simulink model "sim1"  (R2020a)
settings: Solver=ode4  StartTime=0.0  StopTime=inf  FixedStep=0.001  RelTol=1e-3
undefined symbols (not defined in the file or in its folder): National_Instruments, PCI
libraries: sldrtlib x3
settings Model: SimulationMode=external  ExtModeTrigDuration=60000  ExtModeArchiveMode=auto  ExtModeArchiveFileName=data  ExtModeArchiveDirName=E:\work\me-clab2\Lab01  ExtModeAddSuffixToVar=on  Creator=me-clab2  LastModifiedBy=me-clab2
settings RTWCC: Description=Simulink Desktop Real-Time  SystemTargetFile=sldrt.tlc  TemplateMakefile=sldrt.tmf  RTWCompilerOptimization=on
settings CodeAppCC: MaxIdLength=95
settings SimulinkDesktopRealTimeCC: TargetPreCompLibLocation=C:\Program Files\MATLAB\R2020a\toolbox\sldrt\lib\win64

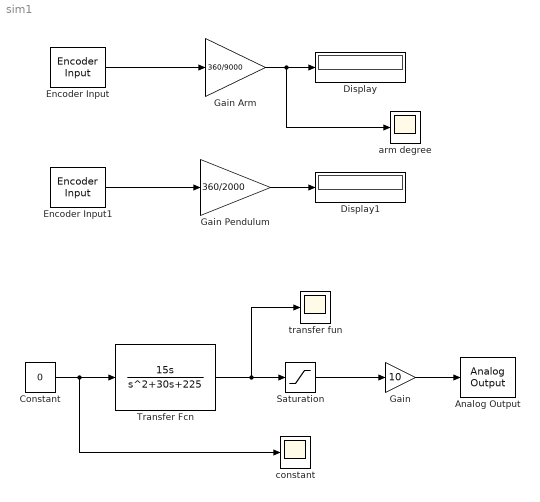
== system sim1 ==
  Analog Output : sldrtlib/Analog Output  SampleTime=0.001  MaxMissedTicks=10  ShowMissedTicks=off  YieldWhenWaiting=off  DrvName=National_Instruments/PCI-6221  DrvAddress=4294967295  DrvOptions=[0 0 0 2 2]  Channels=[2]  RangeMode=1  VoltRange=1  InitialValue=0  FinalValue=0
      settings: AttributesFormatString=National Instruments\nPCI-6221 [auto]
  Constant : Constant  Value=0
  Display : Display
  Display1 : Display
  Encoder Input : sldrtlib/Encoder Input  SampleTime=0.001  MaxMissedTicks=10  ShowMissedTicks=off  YieldWhenWaiting=off  DrvName=National_Instruments/PCI-6221  DrvAddress=4294967295  DrvOptions=[0 0 0 2 2]  Channels=[1]  QuadMode=3  IndexPulse=1  InputFilter=Inf  DataType=1
      settings: AttributesFormatString=National Instruments\nPCI-6221 [auto]
  Encoder Input1 : sldrtlib/Encoder Input  SampleTime=0.001  MaxMissedTicks=10  ShowMissedTicks=off  YieldWhenWaiting=off  DrvName=National_Instruments/PCI-6221  DrvAddress=4294967295  DrvOptions=[0 0 0 2 2]  Channels=[2]  QuadMode=3  IndexPulse=1  InputFilter=Inf  DataType=1
      settings: AttributesFormatString=National Instruments\nPCI-6221 [auto]
  Gain : Gain  Gain=10
  Gain Arm : Gain  Gain=360/9000
  Gain Pendulum : Gain  Gain=360/2000
  Saturation : Saturate  UpperLimit=1  LowerLimit=-1
  Transfer Fcn : TransferFcn  Numerator=[15 0]  Denominator=[1 30 225]
  arm degree : Scope
  constant : Scope
  transfer fun : Scope
  wires:
  Encoder Input/1 -> Gain Arm/1
  Encoder Input1/1 -> Gain Pendulum/1
  Gain Arm/1 -> arm degree/1, Display/1
  Gain Pendulum/1 -> Display1/1
  Constant/1 -> constant/1, Transfer Fcn/1
  Transfer Fcn/1 -> transfer fun/1, Saturation/1
  Saturation/1 -> Gain/1
  Gain/1 -> Analog Output/1
